simulink model "nonlinear"  (R2024b)
settings: Solver=ode4  StartTime=0.0  StopTime=simulation_time  FixedStep=sample_time  RelTol=1e-3
values from neighbouring files (symbols this model uses):
  init_X = initial(i).init_X    [Step3_UAV_altitude.m]    (also in Step3_nonlinear.m)
settings Model: Creator=zhes  LastModifiedBy=zhes

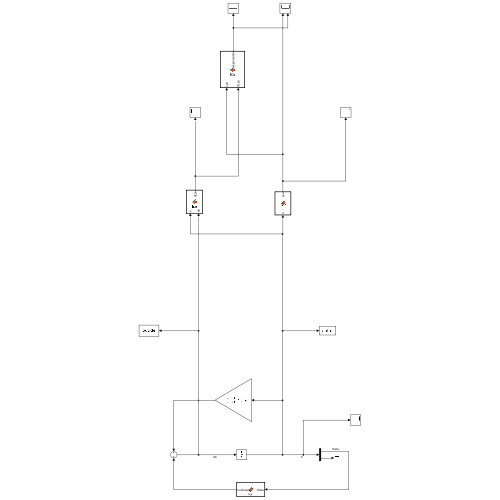
[thumbnail: Simulink's stored preview of the top-level diagram]
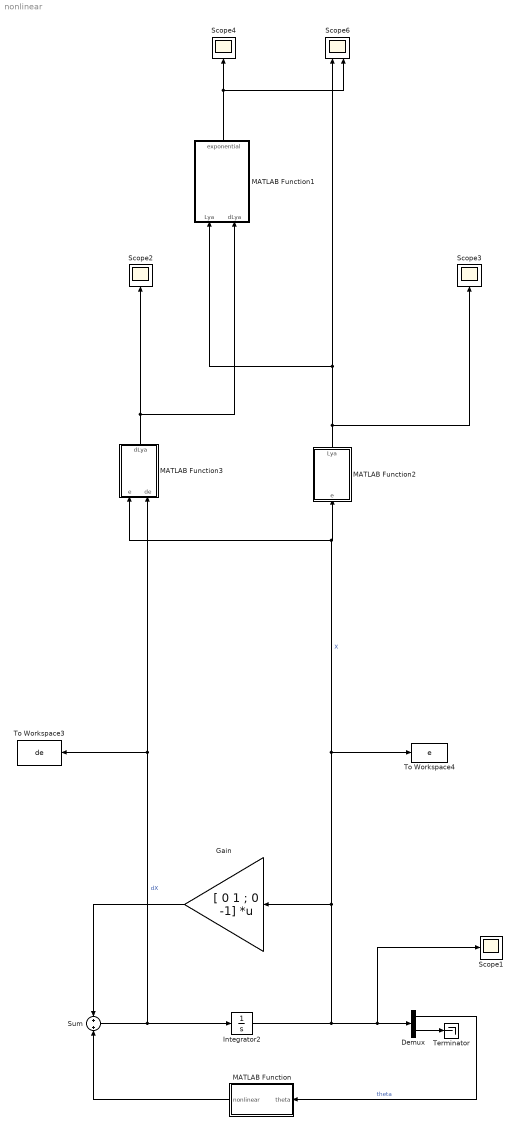
== system nonlinear ==
  Demux : Demux  Outputs=2
  Gain : Gain  Gain="[ 0  1 ;  0  -1]"  Multiplication=Matrix(K*u) (u vector)
  Integrator2 : Integrator  InitialCondition=init_X
  MATLAB Function : MATLAB Function  TreatAsAtomicUnit=on
  MATLAB Function1 : MATLAB Function  TreatAsAtomicUnit=on
  MATLAB Function2 : MATLAB Function  TreatAsAtomicUnit=on
  MATLAB Function3 : MATLAB Function  TreatAsAtomicUnit=on
  Scope{1..4} (4 alike) : Scope
  Scope6 : Scope  NumInputPorts=2
  Sum : Sum  Inputs=+|+
  Terminator : Terminator
  To Workspace3 : ToWorkspace  VariableName=de  SaveFormat=Structure With Time  SampleTime=-1
  To Workspace4 : ToWorkspace  VariableName=e  SaveFormat=Structure With Time  SampleTime=-1
  wires:
  MATLAB Function1/1(exponential) -> Scope6/2, Scope4/1
  MATLAB Function2/1(Lya) -> MATLAB Function1/1(Lya), Scope6/1, Scope3/1
  MATLAB Function3/1(dLya) -> MATLAB Function1/2(dLya), Scope2/1
  Integrator2/1 -> Scope1/1, Demux/1, Gain/1, MATLAB Function3/1(e), MATLAB Function2/1(e), To Workspace4/1  "X"
  Sum/1 -> Integrator2/1, To Workspace3/1, MATLAB Function3/2(de)  "dX"
  Gain/1 -> Sum/1
  Demux/1 -> MATLAB Function/1(theta)  "theta"
  Demux/2 -> Terminator/1
  MATLAB Function/1(nonlinear) -> Sum/2

== matlab function nonlinear/MATLAB Function ==
  data: theta input; nonlinear output
function nonlinear = fcn(theta)

nonlinear = [0 ; -sin(theta)];

== matlab function nonlinear/MATLAB Function2 ==
  data: e input; Lya output
function Lya = fcn(e)

A = [ 0.511472675172699   0.435836007038090
   0.435836007038090   0.378094887153988 ]; % lambda = 1.5

Lya = e.' * A * e;

== matlab function nonlinear/MATLAB Function3 ==
  data: e input; dLya output; de input
function dLya = fcn(e, de)

de1 = e(1);
de2 = e(2);

dde1 = de(1);
dde2 = de(2);


A = [ 0.511472675172699   0.435836007038090
   0.435836007038090   0.378094887153988 ]; % lambda = 1.5

dLya = de' * A * e + e' * A * de;

== matlab function nonlinear/MATLAB Function1 ==
  data: Lya input; exponential output; dLya input
function exponential = fcn(Lya, dLya)

lambda = 1.5;

exponential = dLya + lambda * Lya;
